simulink model "robot"  (R2024a)
settings: Solver=FixedStepAuto  StartTime=0.0  StopTime=20  FixedStep=0.01  RelTol=1e-3
libraries: fuzblock x3
settings Model: Creator=VKIST  LastModifiedBy=TRUONG GIANG
settings DebuggingCC: UnconnectedInputMsg=warning  UnconnectedOutputMsg=warning  UnconnectedLineMsg=warning
settings ModelReferenceCC: EnableRefExpFcnMdlSchedulingChecks=on
settings RTWCC: GPUComputeCapability=3.5  DLArmComputeVersion=19.05

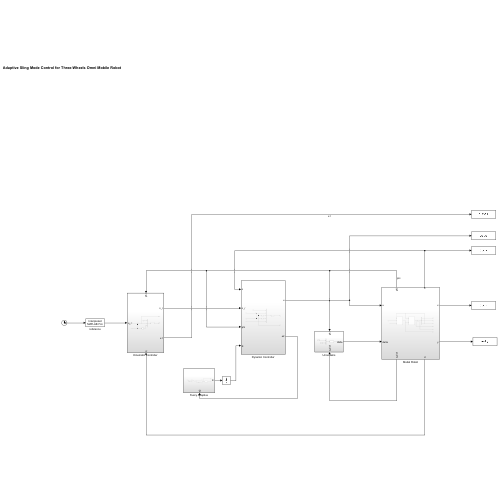
[thumbnail: Simulink's stored preview of the top-level diagram]
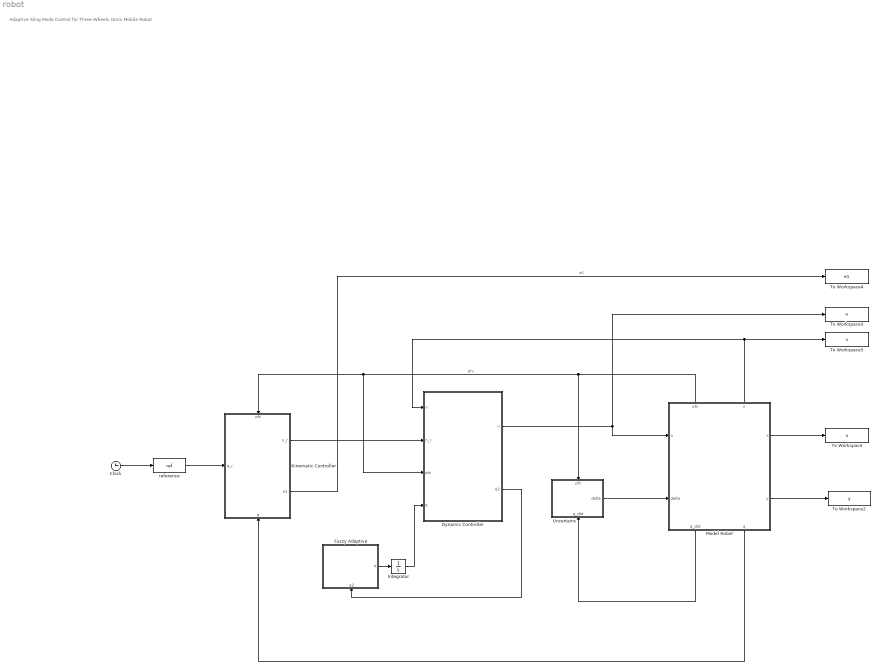
== system robot ==
  note: Adaptive Sling Mode Control for Three-Wheels Omni Mobile Robot
  Clock : Clock
      settings: Decimation=20
  Dynamic Controller : Subsystem
  Fuzzy Adaptive : Subsystem
      settings: PortSchema="{\"entries\":[{\"content\":{\"sides\":[{\"content\":{\"connectorIds\":[]},\"type\":\"ConnectorPlacement.EquallySpacedRectSide\",\"uuid\":\"1d4b4c94-c96b-40bb-9bf0-5078903cdb26\"},{\"content\":{\"connectorIds\":[\"Out1\"],\"side\":\"RIGHT\"},\"type\":\"ConnectorPlacement.EquallySpacedRectSide\",\"uuid\":\"81efdda9-b1ec-4f14-ad93-1b06e88766c1\"},{\"content\":{\"connectorIds\":[],\"side\":\"TOP\"},\"type\":\"ConnectorPlacement.EquallySpacedRectSide\",\"uuid\":\"38e85771-34ed-41c4-8a95-1de5bcf96228\"},{\"content\":{\"connectorIds\":[\"In1\"],\"side\":\"BOTTOM\"},\"type\":\"ConnectorPlacement.EquallySpacedRectSide\",\"uuid\":\"8ac0bd2d-8e34-4e54-b427-a9b77bf55374\"}]},\"type\":\"ConnectorPlacement.EquallySpacedConnector\",\"uuid\":\"31951a69-aed3-4c7e-9a3d-40ef53758fed\"}],\"packageUris\":[\"http://schema.mathworks.com/mf0/Connector/R2020b\"],\"version\":\"1.0\"}"
  Integrator : Integrator
  Kinematic Controller : Subsystem
      settings: PortSchema="{\"entries\":[{\"content\":{\"sides\":[{\"content\":{\"connectorIds\":[\"In1\"]},\"type\":\"ConnectorPlacement.EquallySpacedRectSide\",\"uuid\":\"a14dc590-64b2-4f98-bd89-d061b749c197\"},{\"content\":{\"connectorIds\":[\"Out1\",\"Out2\"],\"side\":\"RIGHT\"},\"type\":\"ConnectorPlacement.EquallySpacedRectSide\",\"uuid\":\"120044c5-80d8-400b-b941-bd8bbb0d305d\"},{\"content\":{\"connectorIds\":[\"In2\"],\"side\":\"TOP\"},\"type\":\"ConnectorPlacement.EquallySpacedRectSide\",\"uuid\":\"4e92235f-f32e-4542-8c0b-731401590a54\"},{\"content\":{\"connectorIds\":[\"In3\"],\"side\":\"BOTTOM\"},\"type\":\"ConnectorPlacement.EquallySpacedRectSide\",\"uuid\":\"e9792b77-5354-4de0-b46b-cfcad6d65c1b\"}]},\"type\":\"ConnectorPlacement.EquallySpacedConnector\",\"uuid\":\"29cb407e-4936-4c7b-888d-e5c07e8ae67c\"}],\"packageUris\":[\"http://schema.mathworks.com/mf0/Connector/R2020b\"],\"version\":\"1.0\"}"
  Model Robot : Subsystem
      settings: PortSchema="{\"entries\":[{\"content\":{\"sides\":[{\"content\":{\"connectorIds\":[\"In1\",\"In2\"]},\"type\":\"ConnectorPlacement.EquallySpacedRectSide\",\"uuid\":\"31b5d89e-c3f9-4f7c-9392-228f8c60e74e\"},{\"content\":{\"connectorIds\":[\"Out1\",\"Out2\"],\"side\":\"RIGHT\"},\"type\":\"ConnectorPlacement.EquallySpacedRectSide\",\"uuid\":\"51f31039-403a-4d76-81cb-a4afb053ddda\"},{\"content\":{\"connectorIds\":[\"Out5\",\"Out6\"],\"side\":\"TOP\"},\"type\":\"ConnectorPlacement.EquallySpacedRectSide\",\"uuid\":\"1e22faa2-b3a5-4107-a2e4-94a4f7f360ea\"},{\"content\":{\"connectorIds\":[\"Out3\",\"Out4\"],\"side\":\"BOTTOM\"},\"type\":\"ConnectorPlacement.EquallySpacedRectSide\",\"uuid\":\"f33b42ed-31c7-4037-aba6-cfe2508847b2\"}]},\"type\":\"ConnectorPlacement.EquallySpacedConnector\",\"uuid\":\"bd468eef-5652-437e-a30a-cca7e1124bc9\"}],\"packageUris\":[\"http://schema.mathworks.com/mf0/Connector/R2020b\"],\"version\":\"1.0\"}"
  To Workspace : ToWorkspace  VariableName=x  SampleTime=-1
  To Workspace2 : ToWorkspace  VariableName=y  SampleTime=-1
  To Workspace3 : ToWorkspace  VariableName=u  SampleTime=-1
  To Workspace4 : ToWorkspace  VariableName=e1  SampleTime=-1
  To Workspace5 : ToWorkspace  VariableName=v  SampleTime=-1
  Uncertains : Subsystem
      settings: PortSchema="{\"entries\":[{\"content\":{\"sides\":[{\"content\":{\"connectorIds\":[]},\"type\":\"ConnectorPlacement.EquallySpacedRectSide\",\"uuid\":\"aba4cdb2-5240-450a-8f76-bbf8d9357908\"},{\"content\":{\"connectorIds\":[\"Out1\"],\"side\":\"RIGHT\"},\"type\":\"ConnectorPlacement.EquallySpacedRectSide\",\"uuid\":\"0a1c664b-48c3-4c0b-a285-e96212d83945\"},{\"content\":{\"connectorIds\":[\"In1\"],\"side\":\"TOP\"},\"type\":\"ConnectorPlacement.EquallySpacedRectSide\",\"uuid\":\"c2b8caca-ebe9-4e76-a354-25b0f3bba02b\"},{\"content\":{\"connectorIds\":[\"In2\"],\"side\":\"BOTTOM\"},\"type\":\"ConnectorPlacement.EquallySpacedRectSide\",\"uuid\":\"ca5d3511-e150-45c1-9cdc-69981c35d8cc\"}]},\"type\":\"ConnectorPlacement.EquallySpacedConnector\",\"uuid\":\"07857a77-fb41-4f55-909b-92520330f109\"}],\"packageUris\":[\"http://schema.mathworks.com/mf0/Connector/R2020b\"],\"version\":\"1.0\"}"
  reference : MATLABFcn  MATLABFcn=ref  OutputDimensions=3
  wires:
  Clock/1 -> reference/1
  Uncertains/1(delta) -> Model Robot/2(delta)
  Model Robot/5(phi) -> Kinematic Controller/2(phi), Dynamic Controller/3(phi), Uncertains/1(phi)  "phi"
  Model Robot/3(q_dot) -> Uncertains/2(q_dot)
  Dynamic Controller/1(u) -> Model Robot/1(u), To Workspace3/1
  Model Robot/4(q) -> Kinematic Controller/3(q)
  reference/1 -> Kinematic Controller/1(q_r)
  Kinematic Controller/2(e1) -> To Workspace4/1  "e1"
  Dynamic Controller/2(e2) -> Fuzzy Adaptive/1(e2)
  Kinematic Controller/1(n_r) -> Dynamic Controller/2(n_r)
  Model Robot/1(x) -> To Workspace/1
  Model Robot/2(y) -> To Workspace2/1
  Model Robot/6(n) -> Dynamic Controller/1(n), To Workspace5/1
  Fuzzy Adaptive/1(K) -> Integrator/1
  Integrator/1 -> Dynamic Controller/4(K)

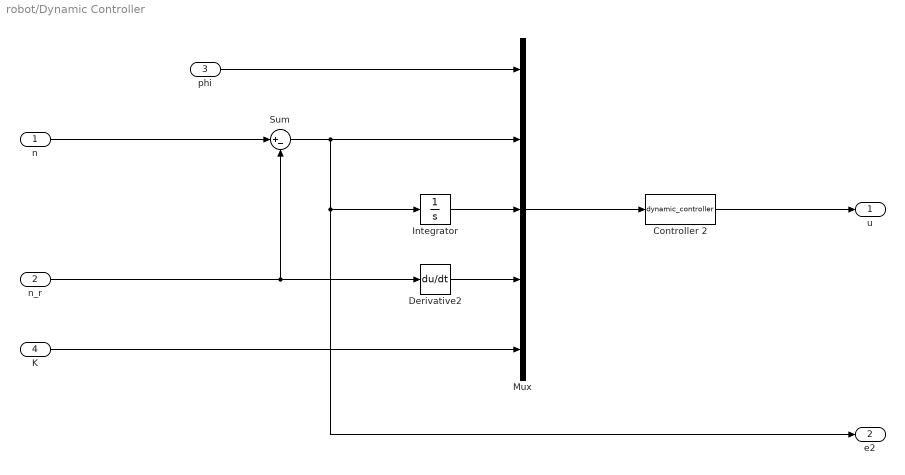
== system robot/Dynamic Controller ==
  n : Inport
  n_r : Inport  Port=2
  phi : Inport  Port=3
  K : Inport  Port=4
  Controller 2 : MATLABFcn  MATLABFcn=dynamic_controller  OutputDimensions=3
  Derivative2 : Derivative
  Integrator : Integrator
  Mux : Mux  Inputs=5
  Sum : Sum  Inputs=|+-
  u : Outport
  e2 : Outport  Port=2
  wires:
  Controller 2/1 -> u/1
  phi/1 -> Mux/1
  n/1 -> Sum/1
  n_r/1 -> Sum/2, Derivative2/1
  Mux/1 -> Controller 2/1
  Sum/1 -> e2/1, Integrator/1, Mux/2
  Integrator/1 -> Mux/3
  Derivative2/1 -> Mux/4
  K/1 -> Mux/5

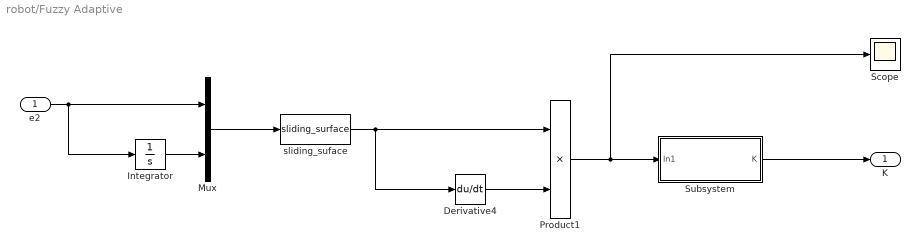
== system robot/Fuzzy Adaptive ==
  e2 : Inport
  Derivative4 : Derivative
  Integrator : Integrator
  Mux : Mux  Inputs=2
  Product1 : Product
  Scope : Scope
  Subsystem : Subsystem
  sliding_suface : MATLABFcn  MATLABFcn=sliding_surface  OutputDimensions=3
  K : Outport
  wires:
  sliding_suface/1 -> Derivative4/1, Product1/1
  Product1/1 -> Scope/1, Subsystem/1(In1)
  Derivative4/1 -> Product1/2
  Mux/1 -> sliding_suface/1
  e2/1 -> Integrator/1, Mux/1
  Subsystem/1(K) -> K/1
  Integrator/1 -> Mux/2

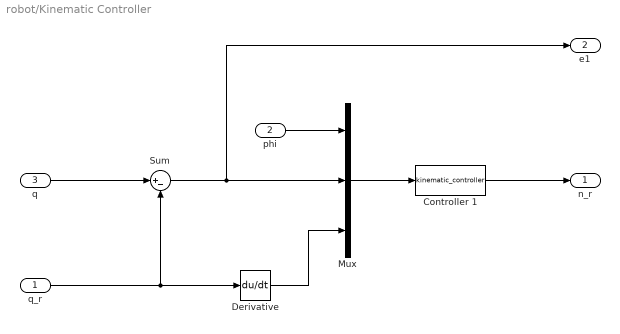
== system robot/Kinematic Controller ==
  q_r : Inport
  phi : Inport  Port=2
  q : Inport  Port=3
  Controller 1 : MATLABFcn  MATLABFcn=kinematic_controller  OutputDimensions=3
  Derivative : Derivative
  Mux : Mux  Inputs=3
  Sum : Sum  Inputs=|+-
  n_r : Outport
  e1 : Outport  Port=2
  wires:
  q_r/1 -> Derivative/1, Sum/2
  q/1 -> Sum/1
  Controller 1/1 -> n_r/1
  Mux/1 -> Controller 1/1
  phi/1 -> Mux/1
  Sum/1 -> Mux/2, e1/1
  Derivative/1 -> Mux/3

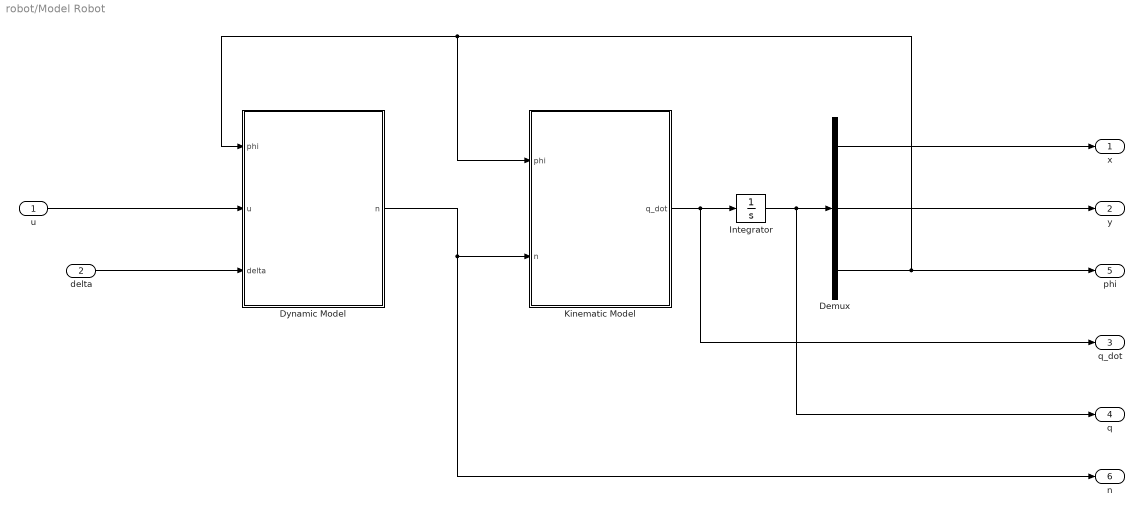
== system robot/Model Robot ==
  u : Inport
  delta : Inport  Port=2
  Demux : Demux  Outputs=3
  Dynamic Model : Subsystem
  Integrator : Integrator
  Kinematic Model : Subsystem
  x : Outport
  y : Outport  Port=2
  q_dot : Outport  Port=3
  q : Outport  Port=4
  phi : Outport  Port=5
  n : Outport  Port=6
  wires:
  Kinematic Model/1(q_dot) -> q_dot/1, Integrator/1
  Integrator/1 -> q/1, Demux/1
  Demux/1 -> x/1
  Demux/2 -> y/1
  Demux/3 -> phi/1, Kinematic Model/1(phi), Dynamic Model/1(phi)
  delta/1 -> Dynamic Model/3(delta)
  u/1 -> Dynamic Model/2(u)
  Dynamic Model/1(n) -> n/1, Kinematic Model/2(n)

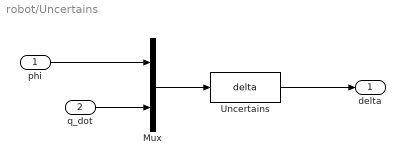
== system robot/Uncertains ==
  phi : Inport
  q_dot : Inport  Port=2
  Mux : Mux  Inputs=2
  Uncertains : MATLABFcn  MATLABFcn=delta  OutputDimensions=3
  delta : Outport
  wires:
  Uncertains/1 -> delta/1
  Mux/1 -> Uncertains/1
  q_dot/1 -> Mux/2
  phi/1 -> Mux/1

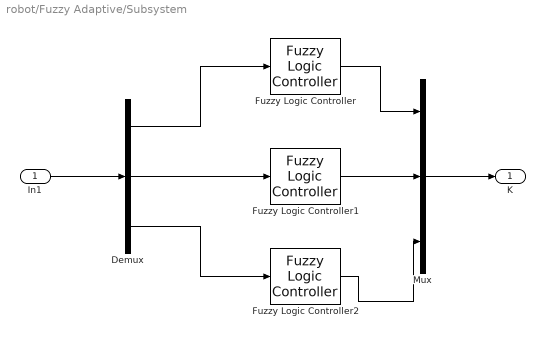
== system robot/Fuzzy Adaptive/Subsystem ==
  In1 : Inport
  Demux : Demux  Outputs=3
  Fuzzy Logic Controller : fuzblock/Fuzzy Logic  Controller  FIS='fuzzy0.fis'  OutputSampleNumber=101  DataType=double  FuzzifiedInputs=off  RuleFiringStrengths=off  RuleOutputs=off  AggregatedOutputs=off  SimulateUsing=Interpreted execution  OutOfRangeInputValueMessage=warning  NoRuleFiredMessage=warning  EmptyOutputFuzzySetMessage=warning
  Fuzzy Logic Controller1 : fuzblock/Fuzzy Logic  Controller  FIS='fuzzy0.fis'  OutputSampleNumber=101  DataType=double  FuzzifiedInputs=off  RuleFiringStrengths=off  RuleOutputs=off  AggregatedOutputs=off  SimulateUsing=Interpreted execution  OutOfRangeInputValueMessage=warning  NoRuleFiredMessage=warning  EmptyOutputFuzzySetMessage=warning
  Fuzzy Logic Controller2 : fuzblock/Fuzzy Logic  Controller  FIS='fuzzy0.fis'  OutputSampleNumber=101  DataType=double  FuzzifiedInputs=off  RuleFiringStrengths=off  RuleOutputs=off  AggregatedOutputs=off  SimulateUsing=Interpreted execution  OutOfRangeInputValueMessage=warning  NoRuleFiredMessage=warning  EmptyOutputFuzzySetMessage=warning
  Mux : Mux  Inputs=3
  K : Outport
  wires:
  Fuzzy Logic Controller1/1 -> Mux/2
  Mux/1 -> K/1
  Fuzzy Logic Controller/1 -> Mux/1
  In1/1 -> Demux/1
  Demux/2 -> Fuzzy Logic Controller1/1
  Demux/1 -> Fuzzy Logic Controller/1
  Demux/3 -> Fuzzy Logic Controller2/1
  Fuzzy Logic Controller2/1 -> Mux/3

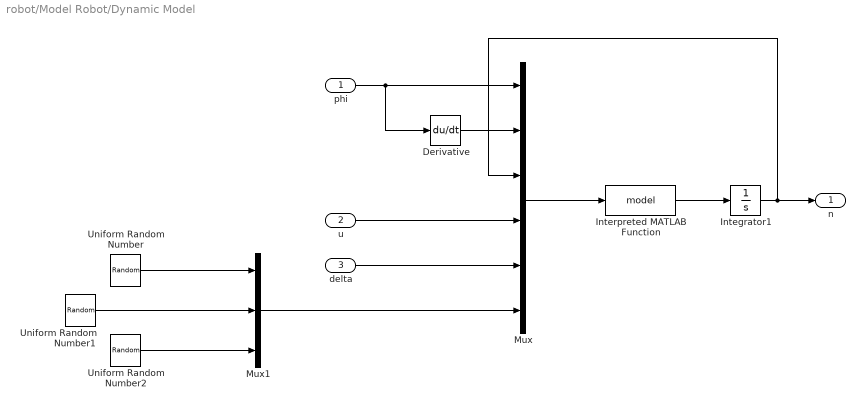
== system robot/Model Robot/Dynamic Model ==
  phi : Inport
  u : Inport  Port=2
  delta : Inport  Port=3
  Derivative : Derivative
  Integrator1 : Integrator
  Interpreted MATLAB Function : MATLABFcn  MATLABFcn=model  OutputDimensions=3
  Mux : Mux  Inputs=6
  Mux1 : Mux  Inputs=3
  Uniform Random Number : UniformRandomNumber  Minimum=-2  Maximum=2  SampleTime=0.1
  Uniform Random Number1 : UniformRandomNumber  Minimum=-2  Maximum=2  SampleTime=0.1
  Uniform Random Number2 : UniformRandomNumber  Minimum=-2  Maximum=2  SampleTime=0.1
  n : Outport
  wires:
  Mux/1 -> Interpreted MATLAB Function/1
  phi/1 -> Mux/1, Derivative/1
  u/1 -> Mux/4
  delta/1 -> Mux/5
  Derivative/1 -> Mux/2
  Interpreted MATLAB Function/1 -> Integrator1/1
  Integrator1/1 -> Mux/3, n/1
  Mux1/1 -> Mux/6
  Uniform Random Number2/1 -> Mux1/3
  Uniform Random Number1/1 -> Mux1/2
  Uniform Random Number/1 -> Mux1/1

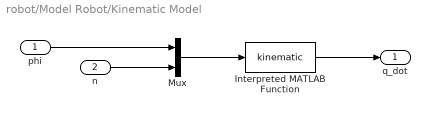
== system robot/Model Robot/Kinematic Model ==
  phi : Inport
  n : Inport  Port=2
  Interpreted MATLAB Function : MATLABFcn  MATLABFcn=kinematic  OutputDimensions=3
  Mux : Mux  Inputs=2
  q_dot : Outport
  wires:
  Mux/1 -> Interpreted MATLAB Function/1
  Interpreted MATLAB Function/1 -> q_dot/1
  phi/1 -> Mux/1
  n/1 -> Mux/2
